simulink model "SaturationAndDeadzoneExample"  (R2019b)
settings: Solver=VariableStepAuto  StartTime=0.0  StopTime=4  RelTol=1e-3
libraries: simulink x1
settings Model: Creator=efrem  LastModifiedBy=Já
settings DataIOCC: ReturnWorkspaceOutputs=off
settings DebuggingCC: ArithmeticOperatorsInVariantConditions=warning
settings SFSimCC: SimUseLocalCustomCode=off  CustomCodeUndefinedFunction=UseInterfaceOnly
settings RTWCC: RTWUseLocalCustomCode=off

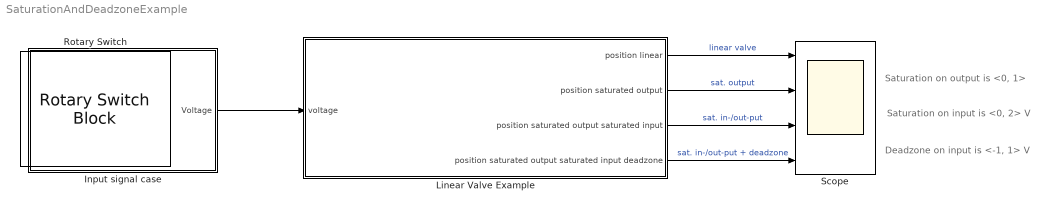
== system SaturationAndDeadzoneExample ==
  note: Saturation on output is <0, 1>
  note: Saturation on input is <0, 2> V
  note: Deadzone on input is <-1, 1> V
  Input signal case : Subsystem  mask{signal_case=1}
      mask prompts: signal_case "Signal type"
  Linear Valve Example : Subsystem
  Rotary Switch : RotarySwitchBlock
      settings: Values={{'Ramp', '0.5 V', '1.5 V', '3 V'}, [1 2 3 4]}
  Scope : Scope  NumInputPorts=4
  wires:
  Linear Valve Example/1(position linear) -> Scope/1  "linear valve"
  Linear Valve Example/2(position saturated output) -> Scope/2  "sat. output"
  Linear Valve Example/3(position saturated output saturated input) -> Scope/3  "sat. in-/out-put"
  Linear Valve Example/4(position saturated output saturated input deadzone) -> Scope/4  "sat. in-/out-put + deadzone"
  Input signal case/1(Voltage) -> Linear Valve Example/1("voltage ")

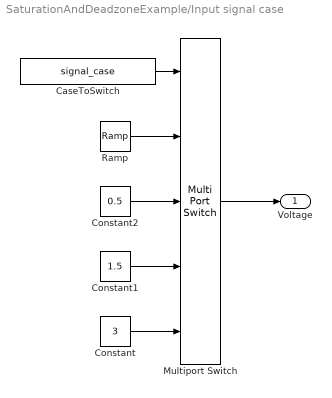
== system SaturationAndDeadzoneExample/Input signal case ==
  CaseToSwitch : Constant  Value=signal_case
  Constant : Constant  Value=3
  Constant1 : Constant  Value=1.5
  Constant2 : Constant  Value=0.5
  Multiport Switch : MultiPortSwitch  Inputs=4
  Ramp : simulink/Sources/Ramp  slope=2  start=0  InitialOutput=0
  Voltage : Outport  VectorParamsAs1DForOutWhenUnconnected=off
  wires:
  Constant2/1 -> Multiport Switch/3
  Constant/1 -> Multiport Switch/5
  Constant1/1 -> Multiport Switch/4
  CaseToSwitch/1 -> Multiport Switch/1
  Multiport Switch/1 -> Voltage/1
  Ramp/1 -> Multiport Switch/2

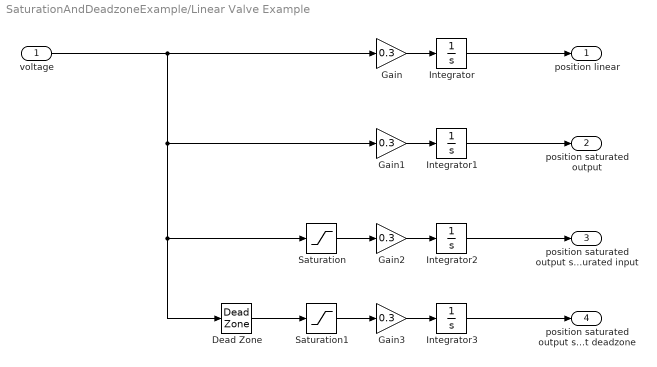
== system SaturationAndDeadzoneExample/Linear Valve Example ==
  "voltage " : Inport
  Dead Zone : DeadZone  LowerValue=-1  UpperValue=1
  Gain{,1..3} (4 alike) : Gain  Gain=0.3
  Integrator : Integrator
  Integrator1 : Integrator  LimitOutput=on  UpperSaturationLimit=1  LowerSaturationLimit=0
  Integrator2 : Integrator  LimitOutput=on  UpperSaturationLimit=1  LowerSaturationLimit=0
  Integrator3 : Integrator  LimitOutput=on  UpperSaturationLimit=1  LowerSaturationLimit=0
  Saturation : Saturate  UpperLimit=2  LowerLimit=0
  Saturation1 : Saturate  UpperLimit=2  LowerLimit=0
  position linear : Outport  VectorParamsAs1DForOutWhenUnconnected=off
  position saturated output : Outport  Port=2  VectorParamsAs1DForOutWhenUnconnected=off
  position saturated output saturated input : Outport  Port=3  VectorParamsAs1DForOutWhenUnconnected=off
  position saturated output saturated input deadzone : Outport  Port=4  VectorParamsAs1DForOutWhenUnconnected=off
  wires:
  Integrator/1 -> position linear/1
  Saturation/1 -> Gain2/1
  Saturation1/1 -> Gain3/1
  Integrator1/1 -> position saturated output/1
  Integrator2/1 -> position saturated output saturated input/1
  "voltage "/1 -> Gain1/1, Dead Zone/1, Saturation/1, Gain/1
  Integrator3/1 -> position saturated output saturated input deadzone/1
  Gain/1 -> Integrator/1
  Gain1/1 -> Integrator1/1
  Gain2/1 -> Integrator2/1
  Gain3/1 -> Integrator3/1
  Dead Zone/1 -> Saturation1/1
